simulink model "unsupervised_controller"  (R2016a)
settings: Solver=FixedStepAuto  StartTime=0.0  StopTime=30  FixedStep=0.01  MaxStep=0.01  RelTol=1e-3
model workspace (MAT data in the model file):
  c = 1
  k = 2
  m = 3
settings Model: Creator=The MathWorks, Inc.  LastModifiedBy=Hamid
settings DataIOCC: LimitDataPoints=on  SaveFormat=Array  SignalLogging=off
settings DebuggingCC: AllowSymbolicDim=off
settings HardwareCC: ProdBitPerPointer=32  ProdLargestAtomicFloat=None  ProdIntDivRoundTo=Undefined  ProdEndianess=Unspecified  ProdWordSize=32  ProdHWDeviceType=32-bit Generic
settings ModelReferenceCC: PropagateSignalLabelsOutOfModel=off
settings ConfigComp: CovModelRefEnable=Off

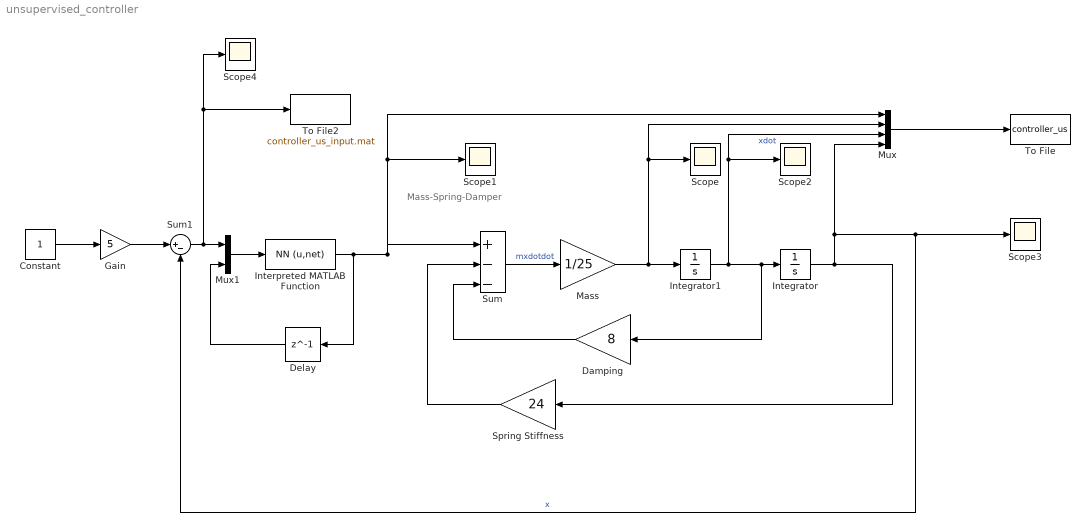
== system unsupervised_controller ==
  note: Mass-Spring-Damper
  Constant : Constant
  Damping : Gain  Gain=8
  Delay : Delay  DelayLength=1
  Gain : Gain  Gain=5
  Integrator : Integrator
  Integrator1 : Integrator  InitialCondition=2.4803
  Interpreted MATLAB Function : MATLABFcn  MATLABFcn=NN (u,net)
  Mass : Gain  Gain=1/25
  Mux : Mux
  Mux1 : Mux  Inputs=2
  Scope{,1..4} (5 alike) : Scope
  Spring Stiffness : Gain  Gain=24
  Sum : Sum  Inputs=|+--
  Sum1 : Sum  Inputs=|+-
  To File : ToFile  Filename=controller_us  MatrixName=controller_us  SaveFormat=Timeseries
  To File2 : ToFile  Filename=controller_us_input.mat  MatrixName=controller_us_input  SaveFormat=Timeseries
  wires:
  Integrator/1 -> Scope3/1, Sum1/2, Mux/4, Spring Stiffness/1  "x"
  Integrator1/1 -> Scope2/1, Mux/3, Integrator/1, Damping/1  "xdot"
  Damping/1 -> Sum/3
  Spring Stiffness/1 -> Sum/2
  Sum/1 -> Mass/1  "mxdotdot"
  Mass/1 -> Scope/1, Mux/2, Integrator1/1
  Mux/1 -> To File/1
  Constant/1 -> Gain/1
  Gain/1 -> Sum1/1
  Sum1/1 -> Mux1/1, Scope4/1, To File2/1
  Interpreted MATLAB Function/1 -> Delay/1, Mux/1, Scope1/1, Sum/1
  Mux1/1 -> Interpreted MATLAB Function/1
  Delay/1 -> Mux1/2
